simulink model "attitude_control"  (R2022b)
settings: Solver=ode45  StartTime=0.0  StopTime=6000  MaxStep=0.01  MinStep=0.001  RelTol=1e-9
values from neighbouring files (symbols this model uses):
  AngularRate_CMD = [0;0;0]    [constant.m]
  Inertia = [0.748 0 0;0 0.793 0;0 0 0.056]    [constant.m]
  invJ_motor = 1/J_motor    (= 20525.4515599)    [constant.m]
  J_motor = 4.872e-5    (= 4.872e-05)    [constant.m]
  Kd = 0.05    [constant.m]
  Ki = 0.01    [constant.m]
  Kp = 0.05    [constant.m]
  Kt = 4.09e-2    (= 0.0409)    [constant.m]
  Li = Kp/Kd*omega_max    (= 837.758)    [constant.m]
  mu = 3.986004418e14    (= 398600441800000)    [constant.m]
  Quat_CMD = [0;0;0;1]    [constant.m]
  rStart = [667939.697348344,-668636.867056020,6906138.58791143]    [constant.m]
  vStart = [-5347.33088536670,-5347.33086786344,-9.04399221326457e-05]    [constant.m]
settings Model: Creator=YJJKDS  LastModifiedBy=yjjkd
settings SolverCC: InitialStep=0.001  AlgebraicLoopSolver=TrustRegion
settings DebuggingCC: UnconnectedInputMsg=warning  UnconnectedOutputMsg=warning  UnconnectedLineMsg=warning  SFMachineParentedDataDiag=warning
settings ModelReferenceCC: EnableRefExpFcnMdlSchedulingChecks=on
settings RTWCC: DLArmComputeVersion=19.05

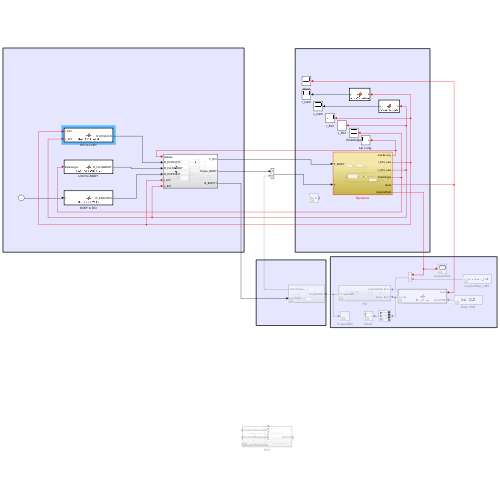
[thumbnail: Simulink's stored preview of the top-level diagram]
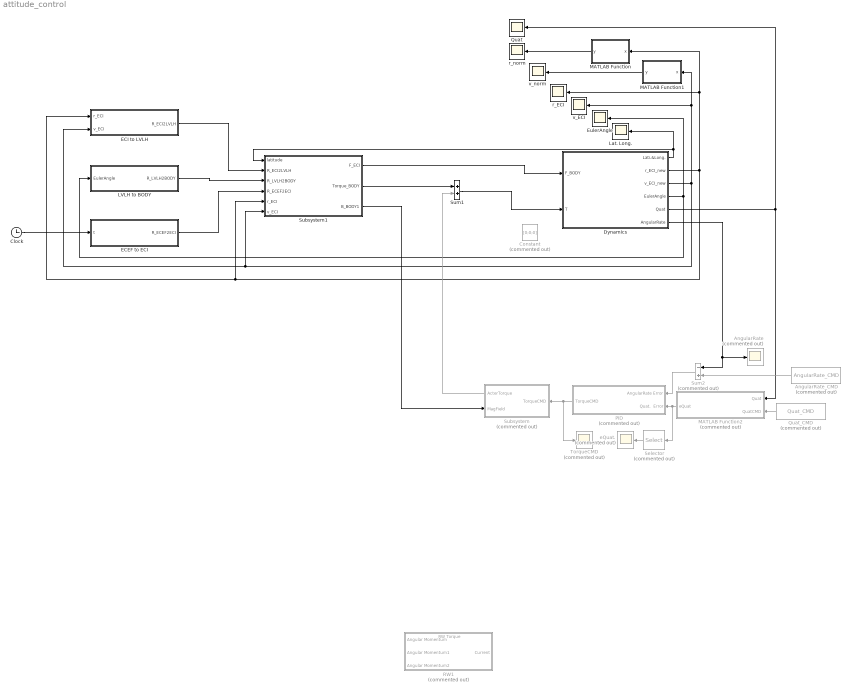
== system attitude_control ==
  AngularRate : Scope  Commented=on
  AngularRate_CMD : Constant  Commented=on  Value=AngularRate_CMD  VectorParams1D=off
  Clock : Clock
  Constant : Constant  Commented=on  Value=[0;0;0]
  Dynamics : Subsystem
  ECEF to ECI : MATLAB Function  TreatAsAtomicUnit=on
  ECI to LVLH : MATLAB Function  TreatAsAtomicUnit=on
  EulerAngle : Scope
  LVLH to BODY : MATLAB Function  TreatAsAtomicUnit=on
  Lat. Long. : Scope
  MATLAB Function : MATLAB Function  TreatAsAtomicUnit=on
  MATLAB Function1 : MATLAB Function  TreatAsAtomicUnit=on
  MATLAB Function2 : MATLAB Function  Commented=on  TreatAsAtomicUnit=on
  PID : Subsystem  Commented=on
  Quat : Scope
  Quat_CMD : Constant  Commented=on  Value=Quat_CMD  VectorParams1D=off
  RW1 : Subsystem  Commented=on
      settings: PortSchema="{\"entries\":[{\"content\":{\"sides\":[{\"content\":{\"connectorIds\":[\"In1\"]},\"type\":\"ConnectorPlacement.EquallySpacedRectSide\",\"uuid\":\"d154d138-04e2-4d68-9401-1b5077d85d63\"},{\"content\":{\"connectorIds\":[\"Out1\",\"Out2\",\"Out3\"],\"side\":\"RIGHT\"},\"type\":\"ConnectorPlacement.EquallySpacedRectSide\",\"uuid\":\"db7db822-5fb9-43df-a7e9-a2adbd254094\"},{\"content\":{\"connectorIds\":[\"Out4\"],\"side\":\"TOP\"},\"type\":\"ConnectorPlacement.EquallySpacedRectSide\",\"uuid\":\"aec92321-89de-4da0-be6a-3b79eff940c1\"},{\"content\":{\"connectorIds\":[],\"side\":\"HIDDEN\"},\"type\":\"ConnectorPlacement.EquallySpacedRectSide\",\"uuid\":\"8cde0229-5647-4a98-afab-a7a8dd712b48\"}]},\"type\":\"ConnectorPlacement.EquallySpacedConnector\",\"uuid\":\"589fcd62-9660-4f9c-92dc-edfb0809d634\"}],\"packageUris\":[\"http://schema.mathworks.com/mf0/Connector/R2020b\"],\"version\":\"1.0\"}"
  Selector : Selector  Commented=on  InputPortWidth=4  IndexOptions=Index vector (dialog)  Indices=[1 2 3]  OutputSizes=1
  Subsystem : Subsystem  Commented=on
      settings: PortSchema="{\"entries\":[{\"content\":{\"sides\":[{\"content\":{\"connectorIds\":[\"In1\"]},\"type\":\"ConnectorPlacement.EquallySpacedRectSide\",\"uuid\":\"9ae17ed7-8875-4cd4-b2e5-a3c4a2531898\"},{\"content\":{\"connectorIds\":[\"Out1\",\"In2\"],\"side\":\"RIGHT\"},\"type\":\"ConnectorPlacement.EquallySpacedRectSide\",\"uuid\":\"80e15e8d-32f1-412a-befc-99fe5fc14d37\"},{\"content\":{\"connectorIds\":[],\"side\":\"TOP\"},\"type\":\"ConnectorPlacement.EquallySpacedRectSide\",\"uuid\":\"8c7ef2c2-210a-4551-a1a8-873a0cff63a6\"},{\"content\":{\"connectorIds\":[],\"side\":\"HIDDEN\"},\"type\":\"ConnectorPlacement.EquallySpacedRectSide\",\"uuid\":\"da26b0ae-0ff8-4760-a8a7-0bcb497aaefe\"}]},\"type\":\"ConnectorPlacement.EquallySpacedConnector\",\"uuid\":\"4a569bc2-6b45-42f2-b88b-6494b0ee63b9\"}],\"packageUris\":[\"http://schema.mathworks.com/mf0/Connector/R2020b\"],\"version\":\"1.0\"}"
  Subsystem1 : Subsystem
  Sum1 : Sum
  Sum2 : Sum  Commented=on  Inputs=-+
  TorqueCMD : Scope  Commented=on
  eQuat. : Scope  Commented=on
  r_ECI : Scope
  r_norm : Scope
  v_ECI : Scope
  v_norm : Scope
  wires:
  Dynamics/3(v_ECI_new) -> Subsystem1/6(v_ECI), ECI to LVLH/2(v_ECI), MATLAB Function1/1(x), v_ECI/1
  Clock/1 -> ECEF to ECI/1(t)
  Dynamics/2(r_ECI_new) -> MATLAB Function/1(x), r_ECI/1, ECI to LVLH/1(r_ECI), Subsystem1/5(r_ECI)
  Dynamics/1(Lati.&Long.) -> Subsystem1/1(latitude), Lat. Long./1
  MATLAB Function/1(y) -> r_norm/1
  MATLAB Function1/1(y) -> v_norm/1
  Dynamics/4(EulerAngle) -> EulerAngle/1, LVLH to BODY/1(EulerAngle)
  Dynamics/5(Quat) -> MATLAB Function2/1(Quat), Quat/1
  Quat_CMD/1 -> MATLAB Function2/2(QuatCMD)
  MATLAB Function2/1(eQuat) -> Selector/1, PID/2(Quat.  Error)
  Dynamics/6(AngularRate) -> Sum2/1, AngularRate/1
  PID/1(TorqueCMD) -> Subsystem/1(TorqueCMD), TorqueCMD/1
  Subsystem/1(ActerTorque) -> Sum1/2
  ECI to LVLH/1(R_ECI2LVLH) -> Subsystem1/2(R_ECI2LVLH)
  LVLH to BODY/1(R_LVLH2BODY) -> Subsystem1/3(R_LVLH2BODY)
  ECEF to ECI/1(R_ECEF2ECI) -> Subsystem1/4(R_ECEF2ECI)
  Subsystem1/2(Torque_BODY) -> Sum1/1
  Subsystem1/1(F_ECI) -> Dynamics/1(F_BODY)
  Subsystem1/3(B_BODY1) -> Subsystem/2(MagField)
  AngularRate_CMD/1 -> Sum2/2
  Sum2/1 -> PID/1(AngularRate Error)
  Selector/1 -> eQuat./1
  Sum1/1 -> Dynamics/2(T)

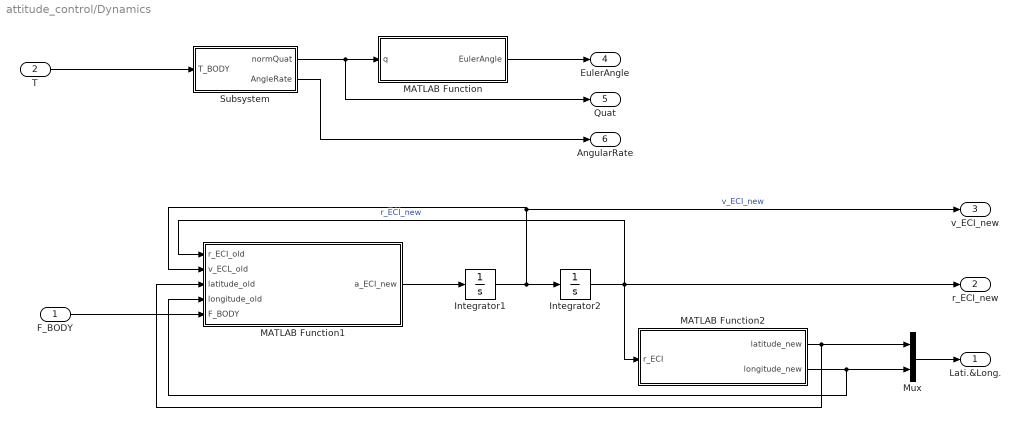
== system attitude_control/Dynamics ==
  F_BODY : Inport
  T : Inport  Port=2
  Integrator1 : Integrator  InitialCondition=vStart
  Integrator2 : Integrator  InitialCondition=rStart
  MATLAB Function : MATLAB Function  TreatAsAtomicUnit=on
  MATLAB Function1 : MATLAB Function  TreatAsAtomicUnit=on
  MATLAB Function2 : MATLAB Function  TreatAsAtomicUnit=on
  Mux : Mux  Inputs=2
  Subsystem : Subsystem
  Lati.&Long. : Outport
  r_ECI_new : Outport  Port=2
  v_ECI_new : Outport  Port=3
  EulerAngle : Outport  Port=4
  Quat : Outport  Port=5
  AngularRate : Outport  Port=6
  wires:
  T/1 -> Subsystem/1(T_BODY)
  MATLAB Function1/1(a_ECI_new) -> Integrator1/1
  Integrator1/1 -> MATLAB Function1/2(v_ECL_old), v_ECI_new/1, Integrator2/1  "v_ECI_new"
  Integrator2/1 -> MATLAB Function1/1(r_ECI_old), r_ECI_new/1, MATLAB Function2/1(r_ECI)  "r_ECI_new"
  F_BODY/1 -> MATLAB Function1/5(F_BODY)
  MATLAB Function2/1(latitude_new) -> Mux/1, MATLAB Function1/3(latitude_old)
  MATLAB Function2/2(longitude_new) -> Mux/2, MATLAB Function1/4(longitude_old)
  Subsystem/1(normQuat) -> Quat/1, MATLAB Function/1(q)
  MATLAB Function/1(EulerAngle) -> EulerAngle/1
  Subsystem/2(AngleRate) -> AngularRate/1
  Mux/1 -> Lati.&Long./1

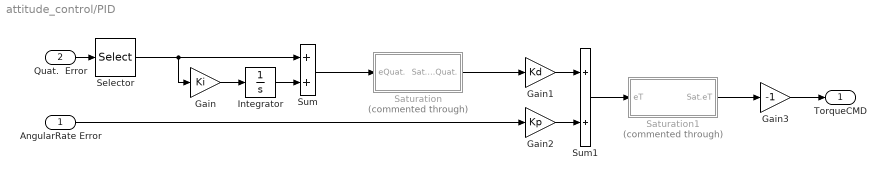
== system attitude_control/PID ==
  AngularRate Error : Inport
  Quat.  Error : Inport  Port=2
  Gain : Gain  Gain=Ki
  Gain1 : Gain  Gain=Kd
  Gain2 : Gain  Gain=Kp
  Gain3 : Gain  Gain=-1
  Integrator : Integrator
  Saturation : Subsystem  Commented=through
  Saturation1 : Subsystem  Commented=through
  Selector : Selector  InputPortWidth=4  IndexOptions=Index vector (dialog)  Indices=[1 2 3]  OutputSizes=1
  Sum : Sum
  Sum1 : Sum
  TorqueCMD : Outport
  wires:
  Integrator/1 -> Sum/2
  Gain/1 -> Integrator/1
  Gain1/1 -> Sum1/1
  Gain2/1 -> Sum1/2
  AngularRate Error/1 -> Gain2/1
  Gain3/1 -> TorqueCMD/1
  Saturation/1(Sat.eQuat.) -> Gain1/1
  Sum1/1 -> Saturation1/1(eT)
  Saturation1/1(Sat.eT) -> Gain3/1
  Sum/1 -> Saturation/1(eQuat.)
  Quat.  Error/1 -> Selector/1
  Selector/1 -> Gain/1, Sum/1

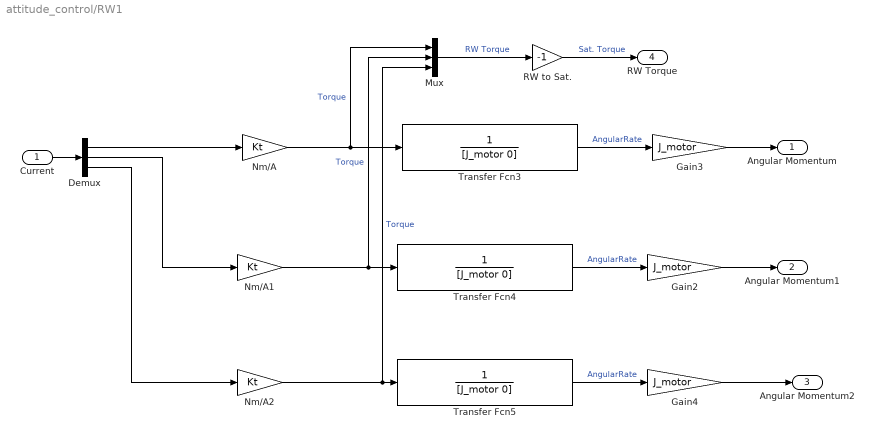
== system attitude_control/RW1 ==
  Current : Inport
  Demux : Demux  Outputs=3
  Gain2 : Gain  Gain=J_motor
  Gain3 : Gain  Gain=J_motor
  Gain4 : Gain  Gain=J_motor
  Mux : Mux  Inputs=3
  Nm/A : Gain  Gain=Kt
  Nm/A1 : Gain  Gain=Kt
  Nm/A2 : Gain  Gain=Kt
  RW to Sat. : Gain  Gain=-1
  Transfer Fcn3 : TransferFcn  Denominator=[J_motor 0]
  Transfer Fcn4 : TransferFcn  Denominator=[J_motor 0]
  Transfer Fcn5 : TransferFcn  Denominator=[J_motor 0]
  Angular Momentum : Outport
  Angular Momentum1 : Outport  Port=2
  Angular Momentum2 : Outport  Port=3
  RW Torque : Outport  Port=4
  wires:
  Transfer Fcn3/1 -> Gain3/1  "AngularRate"
  Gain3/1 -> Angular Momentum/1
  Nm/A/1 -> Mux/1, Transfer Fcn3/1  "Torque"
  Transfer Fcn4/1 -> Gain2/1  "AngularRate"
  Gain2/1 -> Angular Momentum1/1
  Nm/A1/1 -> Mux/2, Transfer Fcn4/1  "Torque"
  Transfer Fcn5/1 -> Gain4/1  "AngularRate"
  Gain4/1 -> Angular Momentum2/1
  Nm/A2/1 -> Mux/3, Transfer Fcn5/1  "Torque"
  Current/1 -> Demux/1
  Demux/1 -> Nm/A/1
  Demux/2 -> Nm/A1/1
  Demux/3 -> Nm/A2/1
  Mux/1 -> RW to Sat./1  "RW Torque"
  RW to Sat./1 -> RW Torque/1  "Sat. Torque"

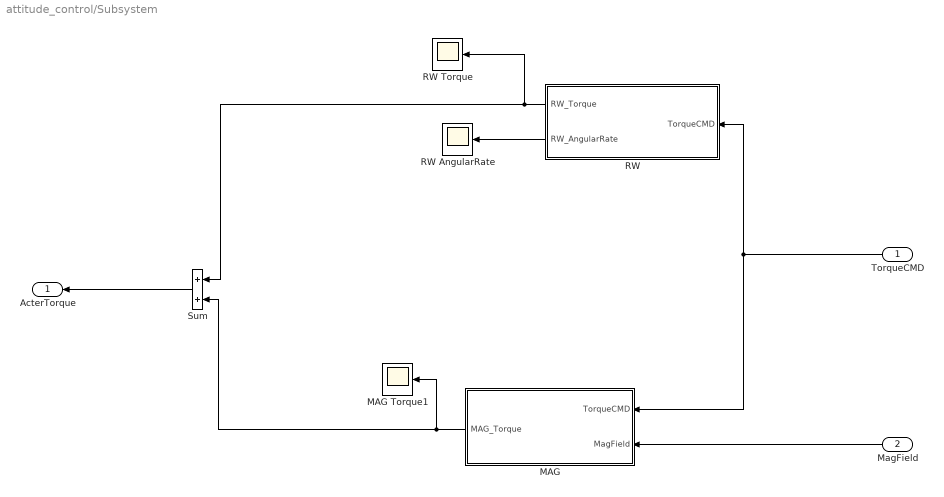
== system attitude_control/Subsystem ==
  TorqueCMD : Inport
  MagField : Inport  Port=2
  MAG : Subsystem
  MAG Torque1 : Scope
  RW : Subsystem
  RW AngularRate : Scope
  RW Torque : Scope
  Sum : Sum
  ActerTorque : Outport
  wires:
  MAG/1(MAG_Torque) -> MAG Torque1/1, Sum/2
  RW/1(RW_Torque) -> Sum/1, RW Torque/1
  RW/2(RW_AngularRate) -> RW AngularRate/1
  Sum/1 -> ActerTorque/1
  MagField/1 -> MAG/2(MagField)
  TorqueCMD/1 -> MAG/1(TorqueCMD), RW/1(TorqueCMD)

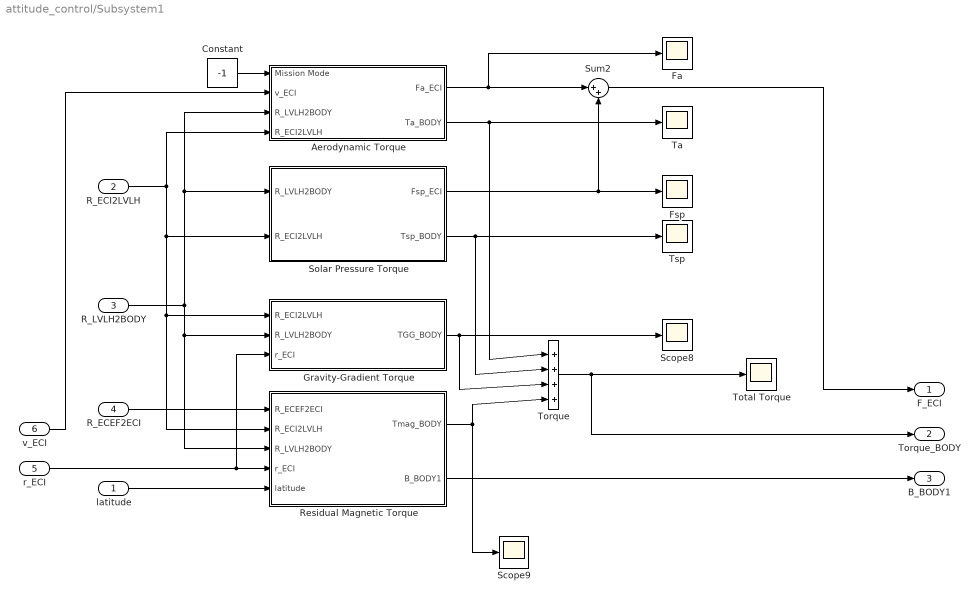
== system attitude_control/Subsystem1 ==
  latitude : Inport
  R_ECI2LVLH : Inport  Port=2
  R_LVLH2BODY : Inport  Port=3
  R_ECEF2ECI : Inport  Port=4
  r_ECI : Inport  Port=5
  v_ECI : Inport  Port=6
  Aerodynamic Torque : Subsystem
  Constant : Constant  Value=-1
  Fa : Scope
  Fsp : Scope
  Gravity-Gradient Torque : Subsystem
  Residual Magnetic Torque : Subsystem
  Scope8 : Scope
  Scope9 : Scope
  Solar Pressure Torque : Subsystem
  Sum2 : Sum  Inputs=|++
  Ta : Scope
  Torque : Sum  Inputs=|++++
  Total Torque : Scope
  Tsp : Scope
  F_ECI : Outport
  Torque_BODY : Outport  Port=2
  B_BODY1 : Outport  Port=3
  wires:
  R_LVLH2BODY/1 -> Aerodynamic Torque/3(R_LVLH2BODY), Solar Pressure Torque/1(R_LVLH2BODY), Residual Magnetic Torque/3(R_LVLH2BODY), Gravity-Gradient Torque/2(R_LVLH2BODY)
  Residual Magnetic Torque/2(B_BODY1) -> B_BODY1/1
  Sum2/1 -> F_ECI/1
  Solar Pressure Torque/2(Tsp_BODY) -> Tsp/1, Torque/2
  latitude/1 -> Residual Magnetic Torque/5(latitude)
  Aerodynamic Torque/2(Ta_BODY) -> Ta/1, Torque/1
  R_ECI2LVLH/1 -> Solar Pressure Torque/2(R_ECI2LVLH), Residual Magnetic Torque/2(R_ECI2LVLH), Gravity-Gradient Torque/1(R_ECI2LVLH), Aerodynamic Torque/4(R_ECI2LVLH)
  r_ECI/1 -> Residual Magnetic Torque/4(r_ECI), Gravity-Gradient Torque/3(r_ECI)
  Constant/1 -> Aerodynamic Torque/1(Mission Mode)
  Gravity-Gradient Torque/1(TGG_BODY) -> Scope8/1, Torque/3
  Solar Pressure Torque/1(Fsp_ECI) -> Fsp/1, Sum2/2
  Residual Magnetic Torque/1(Tmag_BODY) -> Scope9/1, Torque/4
  Torque/1 -> Torque_BODY/1, Total Torque/1
  Aerodynamic Torque/1(Fa_ECI) -> Fa/1, Sum2/1
  v_ECI/1 -> Aerodynamic Torque/2(v_ECI)
  R_ECEF2ECI/1 -> Residual Magnetic Torque/1(R_ECEF2ECI)

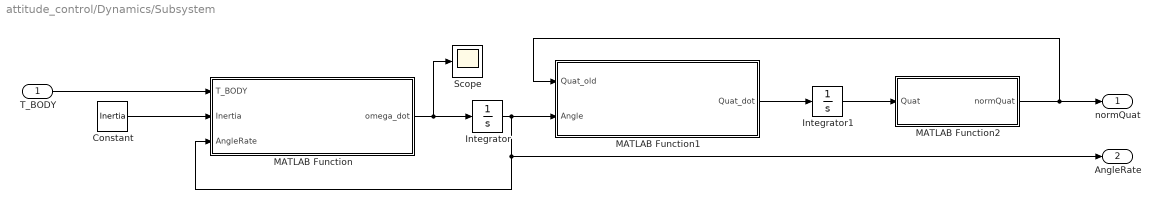
== system attitude_control/Dynamics/Subsystem ==
  T_BODY : Inport
  Constant : Constant  Value=Inertia  VectorParams1D=off
  Integrator : Integrator  InitialCondition=[0;0;0]
  Integrator1 : Integrator  InitialCondition=[1;0;0;0]
  MATLAB Function : MATLAB Function  TreatAsAtomicUnit=on
  MATLAB Function1 : MATLAB Function  TreatAsAtomicUnit=on
  MATLAB Function2 : MATLAB Function  TreatAsAtomicUnit=on
  Scope : Scope
  normQuat : Outport
  AngleRate : Outport  Port=2
  wires:
  T_BODY/1 -> MATLAB Function/1(T_BODY)
  Constant/1 -> MATLAB Function/2(Inertia)
  MATLAB Function/1(omega_dot) -> Scope/1, Integrator/1
  Integrator/1 -> MATLAB Function/3(AngleRate), AngleRate/1, MATLAB Function1/2(Angle)
  MATLAB Function1/1(Quat_dot) -> Integrator1/1
  Integrator1/1 -> MATLAB Function2/1(Quat)
  MATLAB Function2/1(normQuat) -> MATLAB Function1/1(Quat_old), normQuat/1

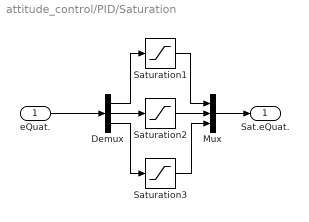
== system attitude_control/PID/Saturation ==
  eQuat. : Inport
  Demux : Demux  Outputs=3
  Mux : Mux  Inputs=3
  Saturation1 : Saturate  UpperLimit=Li  LowerLimit=-Li
  Saturation2 : Saturate  UpperLimit=Li  LowerLimit=-Li
  Saturation3 : Saturate  UpperLimit=Li  LowerLimit=-Li
  Sat.eQuat. : Outport
  wires:
  eQuat./1 -> Demux/1
  Demux/1 -> Saturation1/1
  Demux/2 -> Saturation2/1
  Demux/3 -> Saturation3/1
  Mux/1 -> Sat.eQuat./1
  Saturation2/1 -> Mux/2
  Saturation1/1 -> Mux/1
  Saturation3/1 -> Mux/3

== system attitude_control/PID/Saturation1 ==
  eT : Inport
  Demux : Demux  Outputs=3
  Mux : Mux  Inputs=3
  Saturation : Saturate  UpperLimit=2.3e-3  LowerLimit=-2.3e-3
  Saturation1 : Saturate  UpperLimit=2.3e-3  LowerLimit=-2.3e-3
  Saturation2 : Saturate  UpperLimit=2.3e-3  LowerLimit=-2.3e-3
  Sat.eT : Outport
  wires:
  eT/1 -> Demux/1
  Demux/1 -> Saturation/1
  Demux/2 -> Saturation1/1
  Demux/3 -> Saturation2/1
  Mux/1 -> Sat.eT/1
  Saturation1/1 -> Mux/2
  Saturation/1 -> Mux/1
  Saturation2/1 -> Mux/3

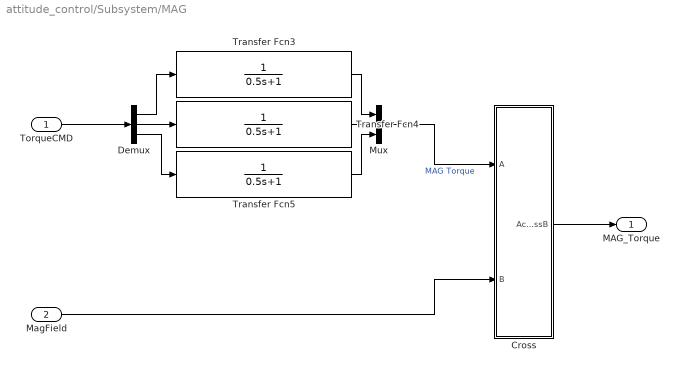
== system attitude_control/Subsystem/MAG ==
  TorqueCMD : Inport
  MagField : Inport  Port=2
  Cross : MATLAB Function  TreatAsAtomicUnit=on
  Demux : Demux  Outputs=3
  Mux : Mux  Inputs=3
  Transfer Fcn3 : TransferFcn  Denominator=[0.5 1]
  Transfer Fcn4 : TransferFcn  Denominator=[0.5 1]
  Transfer Fcn5 : TransferFcn  Denominator=[0.5 1]
  MAG_Torque : Outport
  wires:
  Demux/3 -> Transfer Fcn5/1
  Demux/2 -> Transfer Fcn4/1
  Transfer Fcn3/1 -> Mux/1
  Transfer Fcn5/1 -> Mux/3
  Transfer Fcn4/1 -> Mux/2
  Demux/1 -> Transfer Fcn3/1
  TorqueCMD/1 -> Demux/1
  Mux/1 -> Cross/1(A)  "MAG Torque"
  Cross/1(AcrossB) -> MAG_Torque/1
  MagField/1 -> Cross/2(B)

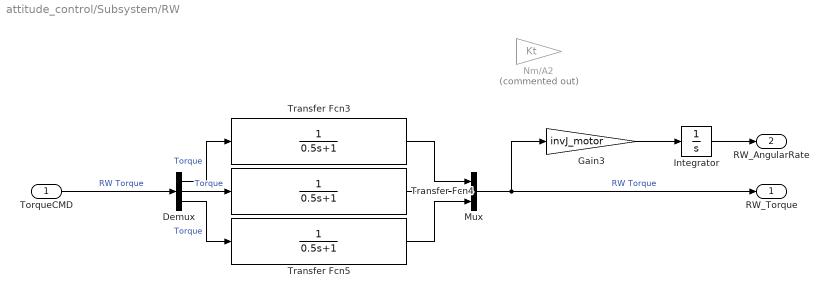
== system attitude_control/Subsystem/RW ==
  TorqueCMD : Inport
  Demux : Demux  Outputs=3
  Gain3 : Gain  Gain=invJ_motor
  Integrator : Integrator  InitialCondition=[0;0;0]
  Mux : Mux  Inputs=3
  Nm/A2 : Gain  Commented=on  Gain=Kt
  Transfer Fcn3 : TransferFcn  Numerator=1  Denominator=[0.5 1]
  Transfer Fcn4 : TransferFcn  Numerator=1  Denominator=[0.5 1]
  Transfer Fcn5 : TransferFcn  Numerator=1  Denominator=[0.5 1]
  RW_Torque : Outport
  RW_AngularRate : Outport  Port=2
  wires:
  Gain3/1 -> Integrator/1
  Integrator/1 -> RW_AngularRate/1
  Demux/1 -> Transfer Fcn3/1  "Torque"
  Transfer Fcn5/1 -> Mux/3
  Demux/2 -> Transfer Fcn4/1  "Torque"
  Transfer Fcn4/1 -> Mux/2
  Demux/3 -> Transfer Fcn5/1  "Torque"
  Transfer Fcn3/1 -> Mux/1
  TorqueCMD/1 -> Demux/1  "RW Torque"
  Mux/1 -> RW_Torque/1, Gain3/1  "RW Torque"

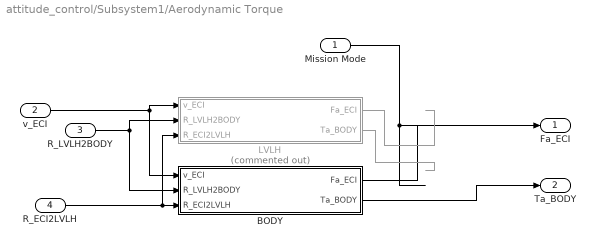
== system attitude_control/Subsystem1/Aerodynamic Torque ==
  Mission Mode : Inport
  v_ECI : Inport  Port=2
  R_LVLH2BODY : Inport  Port=3
  R_ECI2LVLH : Inport  Port=4
  BODY : MATLAB Function  TreatAsAtomicUnit=on
  LVLH : MATLAB Function  Commented=on  TreatAsAtomicUnit=on
  Fa_ECI : Outport
  Ta_BODY : Outport  Port=2
  wires:
  v_ECI/1 -> BODY/1(v_ECI), LVLH/1(v_ECI)
  R_LVLH2BODY/1 -> BODY/2(R_LVLH2BODY), LVLH/2(R_LVLH2BODY)
  Mission Mode/1 -> ?
  R_ECI2LVLH/1 -> LVLH/3(R_ECI2LVLH), BODY/3(R_ECI2LVLH)
  BODY/2(Ta_BODY) -> Ta_BODY/1
  BODY/1(Fa_ECI) -> Fa_ECI/1
  LVLH/1(Fa_ECI) -> ?
  LVLH/2(Ta_BODY) -> ?

== system attitude_control/Subsystem1/Gravity-Gradient Torque ==
  R_ECI2LVLH : Inport
  R_LVLH2BODY : Inport  Port=2
  r_ECI : Inport  Port=3
  Constant : Constant  Value=Inertia  VectorParams1D=off
  Constant1 : Constant  Value=mu
  Gravity Gradient Torque : MATLAB Function  TreatAsAtomicUnit=on
  TGG_BODY : Outport
  wires:
  Gravity Gradient Torque/1(TGG_BODY) -> TGG_BODY/1
  Constant/1 -> Gravity Gradient Torque/2(I)
  Constant1/1 -> Gravity Gradient Torque/3(mu)
  R_LVLH2BODY/1 -> Gravity Gradient Torque/5(R_LVLH2BODY)
  R_ECI2LVLH/1 -> Gravity Gradient Torque/4(R_ECI2LVLH)
  r_ECI/1 -> Gravity Gradient Torque/1(r_ECI)

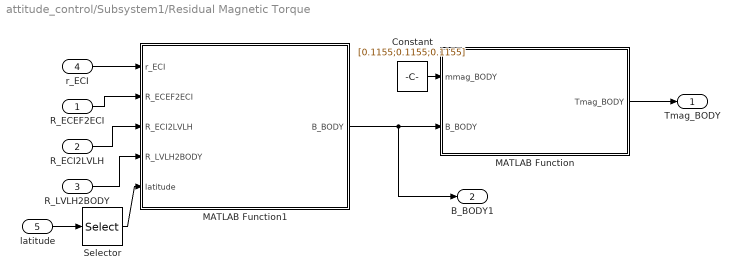
== system attitude_control/Subsystem1/Residual Magnetic Torque ==
  R_ECEF2ECI : Inport
  R_ECI2LVLH : Inport  Port=2
  R_LVLH2BODY : Inport  Port=3
  r_ECI : Inport  Port=4
  latitude : Inport  Port=5
  Constant : Constant  Value=[0.1155;0.1155;0.1155]  VectorParams1D=off
  MATLAB Function : MATLAB Function  TreatAsAtomicUnit=on
  MATLAB Function1 : MATLAB Function  TreatAsAtomicUnit=on
  Selector : Selector  InputPortWidth=2  IndexOptions=Index vector (dialog)  Indices=[1]  OutputSizes=1
  Tmag_BODY : Outport
  B_BODY1 : Outport  Port=2
  wires:
  MATLAB Function1/1(B_BODY) -> B_BODY1/1, MATLAB Function/2(B_BODY)
  MATLAB Function/1(Tmag_BODY) -> Tmag_BODY/1
  r_ECI/1 -> MATLAB Function1/1(r_ECI)
  R_ECEF2ECI/1 -> MATLAB Function1/2(R_ECEF2ECI)
  R_ECI2LVLH/1 -> MATLAB Function1/3(R_ECI2LVLH)
  R_LVLH2BODY/1 -> MATLAB Function1/4(R_LVLH2BODY)
  Constant/1 -> MATLAB Function/1(mmag_BODY)
  Selector/1 -> MATLAB Function1/5(latitude)
  latitude/1 -> Selector/1

== system attitude_control/Subsystem1/Solar Pressure Torque ==
  R_LVLH2BODY : Inport
  R_ECI2LVLH : Inport  Port=2
  MATLAB Function : MATLAB Function  TreatAsAtomicUnit=on
  Fsp_ECI : Outport
  Tsp_BODY : Outport  Port=2
  wires:
  MATLAB Function/2(Tsp_BODY) -> Tsp_BODY/1
  MATLAB Function/1(Fsp_ECI) -> Fsp_ECI/1
  R_LVLH2BODY/1 -> MATLAB Function/1(R_LVLH2BODY)
  R_ECI2LVLH/1 -> MATLAB Function/2(R_ECI2LVLH)

== matlab function attitude_control/MATLAB Function ==
  data: x input; y output
function y = normCaculate(x)
u = norm(x);
y = u;

== matlab function attitude_control/MATLAB Function1 ==
  data: x input; y output
function y = normCaculate(x)
u = norm(x);
y = u;

== matlab function attitude_control/Subsystem1/Solar Pressure Torque/MATLAB Function ==
  data: Fsp_ECI output; R_LVLH2BODY input; R_ECI2LVLH input; Tsp_BODY output
function [Fsp_ECI,Tsp_BODY]  = sunlight(R_LVLH2BODY,R_ECI2LVLH)

%% constant
r_cm2cp = [3.390e-3;-5.642e-3;84.51e-3];
r_panel1 = [281.5e-3;0;168e-3];
r_panel2 = [-281.5e-3;0;168e-3];
Ax = 0.0366;
Ay = 0.0828258;
Az = 0.02263;
Apanel = 0.0366;
Apanel_vec_BODY = [0;0;0.0366];
%A_vec = [Ax;Ay;Az];
sunlight_ECI = [1;0;0];%
P = 4.62e-6;

%% dot
sunlight_BODY = R_LVLH2BODY * R_ECI2LVLH * sunlight_ECI;
X_dot = dot(sunlight_BODY,[1;0;0]);
Y_dot = dot(sunlight_BODY,[0;1;0]);
Z_dot = dot(sunlight_BODY,[0;0;1]);

%% F absorb
Ca = 0.9;%absorb coff.
%Fa_BODY = -P * Ca * X_dot * A_vec;

%% F reflection
Cr = 0.85;%reflection coff.
%Fr_BODY = -2*P * Cr * X_dot^2 * A_vec;

%% F scatter
Cs = 0.1;%scatter coff.
%Fs_BODY = -2/3*P * Cs * X_dot * A_vec;

%% F panel


%% Torque
Fx_BODY = -P*Ax*X_dot*((Ca+Cs)*sunlight_BODY+(2*X_dot*Cr+2/3*Cs)*[1;0;0]);
Fy_BODY = -P*Ax*Y_dot*((Ca+Cs)*sunlight_BODY+(2*Y_dot*Cr+2/3*Cs)*[0;1;0]);
Fz_BODY = -P*Ax*Z_dot*((Ca+Cs)*sunlight_BODY+(2*Z_dot*Cr+2/3*Cs)*[0;0;1]);
%Fbody_BODY = Fa_BODY + Fr_BODY + Fs_BODY;
Fsp_BODY = Fx_BODY + Fy_BODY + Fz_BODY;
Fsp_ECI = R_ECI2LVLH' * R_LVLH2BODY' * Fsp_BODY;
Tsp_BODY = cross(r_cm2cp,Fsp_BODY);
end

== matlab function attitude_control/MATLAB Function2 ==
  data: Quat input; eQuat output; QuatCMD input
function eQuat = ErrorQuat(Quat,QuatCMD)
eQuat = [ QuatCMD(4)  QuatCMD(3) -QuatCMD(2) -QuatCMD(1); ...
         -QuatCMD(3)  QuatCMD(4)  QuatCMD(1) -QuatCMD(2); ...
          QuatCMD(2) -QuatCMD(1)  QuatCMD(4) -QuatCMD(3); ...
          QuatCMD(1)  QuatCMD(2)  QuatCMD(3)  QuatCMD(4)] * Quat;
end

== matlab function attitude_control/Subsystem1/Aerodynamic Torque/BODY ==
  data: Fa_ECI output; v_ECI input; Ta_BODY output; R_LVLH2BODY input; R_ECI2LVLH input
function [Fa_ECI,Ta_BODY]  = StationPointing(v_ECI,R_LVLH2BODY,R_ECI2LVLH)
% input:
%  Velocity in ECI:(1x3)
%  R:(3x3)
% output:
%  airdrag in VehicleFix:FaFix(1x3)

%% constant
CD = 2;
r_cm2cp = [3.390e-3;-5.642e-3;84.51e-3];
r_panel1 = [281.5e-3;0;168e-3];
r_panel2 = [-281.5e-3;0;168e-3];
Rho = 0.000639 / 1000000000;%maxmium density at 600km /% kg/km3 to kg/m3
Ax = 0.0366;
Ay = 0.0828258;
Az = 0.02263;
Apanel = 0.0366;
v = norm(v_ECI);

%% LVLH to BODY
v_LVLH = [v;0;0];
v_Body= R_LVLH2BODY * v_LVLH;

%% F air in Body
Fax_Body = 1/2*CD*Ax*Rho*v_Body(1)*v;
Fay_Body = 1/2*CD*Ay*Rho*v_Body(2)*v;
Faz_Body = 1/2*CD*Az*Rho*v_Body(3)*v;
Fcube_BODY = [Fax_Body;Fay_Body;Faz_Body];

Fpanel = 1/2*CD*Apanel*Rho*v_Body(3)*v;

%% torque in BODY
Tcube_BODY = cross(r_cm2cp,Fcube_BODY);
Tpanel1_BODY = cross(r_panel1-r_cm2cp,[0;0;Fpanel]);
Tpanel2_BODY = cross(r_panel2-r_cm2cp,[0;0;Fpanel]);

Fa_BODY = Fcube_BODY + 2*Fpanel;
Fa_ECI = R_ECI2LVLH' * R_LVLH2BODY' * Fa_BODY;
Ta_BODY = Tcube_BODY + Tpanel1_BODY + Tpanel2_BODY;

end

== matlab function attitude_control/Dynamics/Subsystem/MATLAB Function ==
  data: T_BODY input; omega_dot output; Inertia input; AngleRate input
function omega_dot = Dynamics(T_BODY,Inertia,AngleRate)
%
 %omega_dotX = (T_BODY(1) - (Inertia(2,2)-Inertia(3,3))*AngleRate(2)*AngleRate(3) ...
 %                                      + h_RW(3) * AngleRate(2) - h_RW(2) * AngleRate(3) )/Inertia(1,1);
 %omega_dotY = (T_BODY(2) - (Inertia(3,3)-Inertia(1,1))*AngleRate(3)*AngleRate(1) ...
 %                                      + h_RW(1) * AngleRate(3) - h_RW(3) * AngleRate(1) )/Inertia(2,2);
 %omega_dotZ = (T_BODY(3) - (Inertia(1,1)-Inertia(2,2))*AngleRate(1)*AngleRate(2) ...
 %                                      + h_RW(2) * AngleRate(1) - h_RW(1) * AngleRate(2) )/Inertia(3,3);

% omega_dotX = (T_BODY(1) + (Inertia(2,2)-Inertia(3,3))*AngleRate(2)*AngleRate(3) )/Inertia(1,1);
% omega_dotY = (T_BODY(2) + (Inertia(3,3)-Inertia(1,1))*AngleRate(3)*AngleRate(1) )/Inertia(2,2);
% omega_dotZ = (T_BODY(3) + (Inertia(1,1)-Inertia(2,2))*AngleRate(1)*AngleRate(2) )/Inertia(3,3);
% 
% omega_dot = [omega_dotX;omega_dotY;omega_dotZ];

omega_dot = Inertia\T_BODY;
end

== matlab function attitude_control/Dynamics/Subsystem/MATLAB Function1 ==
  data: Quat_old input; Quat_dot output; Angle input
function Quat_dot = QuaternionAttitude(Quat_old,Angle)
%
Quat_dot = 1/2*[    0       Angle(3)  -Angle(2)  Angle(1); ...
                -Angle(3)      0       Angle(1)  Angle(2); ...
                 Angle(2)  -Angle(1)      0      Angle(3); ...
                -Angle(1)  -Angle(2)  -Angle(3)     0    ;] * Quat_old;
end

== matlab function attitude_control/Dynamics/Subsystem/MATLAB Function2 ==
  data: Quat input; normQuat output
function normQuat = normalization(Quat)

normQuat = Quat / norm(Quat);

end

== matlab function attitude_control/Dynamics/MATLAB Function ==
  data: q input; EulerAngle output
function EulerAngle = Quat2Euler(q)

phi = atan2(2*(q(4)*q(1)+q(2)*q(3)),1-2*(q(1)^2)+q(2)^2);
theta = asin(2*(q(4)*q(2)-q(1)*q(3)));
psi = atan2(2*(q(4)*q(3)+q(1)*q(2)),1-2*(q(2)^2)+q(3)^2);
EulerAngle = [phi;theta;psi];
end

== matlab function attitude_control/Subsystem/MAG/Cross ==
  data: A input; AcrossB output; B input
function AcrossB = fcn(A,B)
AcrossB = cross(A,B);
end

== matlab function attitude_control/Subsystem1/Aerodynamic Torque/LVLH ==
  data: Fa_ECI output; v_ECI input; Ta_BODY output; R_LVLH2BODY input; R_ECI2LVLH input
function [Fa_ECI,Ta_BODY]  = EarthPointing(v_ECI,R_LVLH2BODY,R_ECI2LVLH)
% input:
%  Velocity in ECI:(1x3)
%  R:(3x3)
% output:
%  airdrag in LVLH:(1x3)

%% constant
CD = 2;
Rho = 0.000639 / 1000000000;%kg/km3 to kg/m3  %600km
Ax = 0.0366;
r_cm2cp = [3.390e-3;-5.642e-3;84.51e-3];
v = norm(v_ECI);

%% F air in LVLH
Fax = 1/2*CD*Rho*Ax*v*v;
Fay = 0;
Faz = 0;
Fa_LVLH = [Fax;Fay;Faz];

%% F air in BODY
Fa_BODY= R_LVLH2BODY * Fa_LVLH;
Fa_ECI = R_ECI2LVLH' * Fa_LVLH;

%% torque
Ta_BODY = cross(r_cm2cp,Fa_BODY);
end

== matlab function attitude_control/Subsystem1/Gravity-Gradient Torque/Gravity Gradient Torque ==
  data: r_ECI input; I input; mu input; TGG_BODY output; R_ECI2LVLH input; R_LVLH2BODY input
function TGG_BODY = G_Gradient(r_ECI, I, mu, R_ECI2LVLH, R_LVLH2BODY)

r = norm(r_ECI);
u = r_ECI/r;

TGG_ECI = -3*mu/r^5 * cross(u,I*u);
TGG_BODY = R_LVLH2BODY * R_ECI2LVLH * TGG_ECI;

end

== matlab function attitude_control/LVLH to BODY ==
  data: EulerAngle input; R_LVLH2BODY output
function R_LVLH2BODY = Rot_LVLH2BODY(EulerAngle)

phi = EulerAngle(1);%roll
theta = EulerAngle(2);%pitch
psi = EulerAngle(3);%yaw

R_Yaw = [cos(psi) sin(psi) 0; -sin(psi) cos(psi) 0; 0 0 1];
R_Pitch = [cos(theta) 0 -sin(theta); 0 1 0; sin(theta) 0 cos(theta)];
R_Roll = [1 0 0; 0 cos(phi) sin(phi); 0 -sin(phi) cos(phi)];

R_LVLH2BODY = R_Roll * R_Pitch * R_Yaw;
end

== matlab function attitude_control/ECI to LVLH ==
  data: r_ECI input; R_ECI2LVLH output; v_ECI input
function R_ECI2LVLH = Rot_ECI2LVLH(r_ECI, v_ECI)

%% constant
r = norm(r_ECI);
v = norm(v_ECI);

%% AngularMomentum
hh = cross(r_ECI,v_ECI);
h = norm(hh);

%% Base Vector for LVLH
ez = -r_ECI/r;
ey = -hh/h;
ex = cross(ey,ez);

R_ECI2LVLH = [ex,ey,ez]';
end

== matlab function attitude_control/Subsystem1/Residual Magnetic Torque/MATLAB Function ==
  data: mmag_BODY input; Tmag_BODY output; B_BODY input
function Tmag_BODY = ResidualMagnetism(mmag_BODY,B_BODY)

Tmag_BODY = cross(mmag_BODY,B_BODY);

end

== matlab function attitude_control/Subsystem1/Residual Magnetic Torque/MATLAB Function1 ==
  data: r_ECI input; B_BODY output; R_ECEF2ECI input; R_ECI2LVLH input; R_LVLH2BODY input; latitude input
function B_BODY = DipoleModel(r_ECI, R_ECEF2ECI, R_ECI2LVLH, R_LVLH2BODY,latitude)
%% constant
B0 = 3.12e-5;
r = norm(r_ECI);
normalized_r = r/6371000;

%% magnetic vector
Br = -2*B0/normalized_r^3 * sin(latitude);
Btheta = B0/normalized_r^3 * cos(latitude);
absB = B0/normalized_r^3 * sqrt(1+3*sin(latitude)^2);

B_ECEF = [Br;Btheta;absB];
B_BODY = R_LVLH2BODY * R_ECI2LVLH * R_ECEF2ECI * B_ECEF;
end

== matlab function attitude_control/ECEF to ECI ==
  data: t input; R_ECEF2ECI output
function R_ECEF2ECI = Rot_ECEF2ECI(t)
omega = 7.2921e-05;
R_ECEF2ECI = [ cos(omega*t) sin(omega*t) 0; ...
              -sin(omega*t) cos(omega*t) 0; ...
                    0           0        1];

end

== matlab function attitude_control/Dynamics/MATLAB Function1 ==
  data: r_ECI_old input; a_ECI_new output; v_ECL_old input; latitude_old input; longitude_old input; F_BODY input
function a_ECI_new  = PositionVelocity(r_ECI_old, v_ECL_old, latitude_old, longitude_old, F_BODY)
%% J2 pertubation
mu = 3.986004418e14;
Re = 6371000;
J2 = 1082.6e-6;
r = norm(r_ECI_old);
m = 1;
U = -mu/r * (Re/r)^2 * J2 * (3*sin(latitude_old)^2-1);

%% dynamics
a_ECI_new = -mu/r^3*r_ECI_old + F_BODY/m;

end

== matlab function attitude_control/Dynamics/MATLAB Function2 ==
  data: r_ECI input; latitude_new output; longitude_new output
function [latitude_new,longitude_new] = lat_long(r_ECI)
%% lat. long.
latitude_new = atan2(r_ECI(3),sqrt(r_ECI(1)^2+r_ECI(2)^2) );
longitude_new = asin(r_ECI(2)/sqrt(r_ECI(1)^2 + r_ECI(2)^2));

end
